simulink model "E020_R1_U2_aU_window_from_ideal_iqcot_20260701_144800"  (R2024b)
settings: Solver=VariableStepAuto  StartTime=0.0  StopTime=0.54e-3  MaxStep=5e-9  RelTol=1e-3
undefined symbols (not defined in the file): A_init, A_lower, A_upper, Cout, DCR_L1, DCR_L2, DCR_L3, DCR_L4, E020_Boost_Decay_Rate, E020_CurrentLimit_Guard, E020_FastRequest_Enable, E020_FastRequest_Period, E020_FastRequest_PulseWidth, E020_FastRequest_Window, E020_LateRecoveryGuard_Enable, E020_Settling_Band, E020_TonBoost_Enable, E020_TonBoost_Window, E020_Undershoot_Band, E020_Vref, ESR_C, IdealIQCOT_Enable, IL_adc_counts_per_A, IL_pk_limit_adc_neg, IL_pk_limit_adc_pos, Iload_final, Iload_initial, Iph, Iqcot_enable, kappa_cmd, Kiqcot, Kvc_iqcot, L, Lambda0_iqcot, Lambda_m2, rho_cmd, Ri_iqcot, t_load_step, Tblank, Tdead, Tiqcot_leak, Toff_min, Ton_cmd, Ton_iq_max, Ton_iq_min, Ts_ctrl, Tslot, Tss, Tton_boost_max, Vc_bias_iqcot, Vcot_ramp_amp, Vcot_ramp_enable, Vhys, Vin, Vo_ref
libraries: simulink x29, spsCurrentMeasurementLib x8, spsMosfetLib x8, spsSeriesRLCBranchLib x5, spsVoltageMeasurementLib x5, spsDCVoltageSourceLib x4, spsControlledCurrentSourceLib x1, spsGroundLib x1, spspowerguiLib x1
(part 2 of 2)

== system E020_R1_U2_aU_window_from_ideal_iqcot_20260701_144800/GateDriver_1Phase1/OnDelay1 ==
  u : Inport
  Compare To Constant : simulink/Logic and Bit Operations/Compare To Constant  relop=>=  const=Tdead  OutDataTypeStr=boolean
  Data Type Conversion : DataTypeConversion  OutDataTypeStr=double  SaturateOnIntegerOverflow=off  RndMeth=Floor
  Integrator : Integrator  ExternalReset=level
  Logical Operator : Logic  Operator=NOT  AllPortsSameDT=off  OutDataTypeStr=boolean
  y : Outport
  wires:
  u/1 -> Data Type Conversion/1, Logical Operator/1
  Logical Operator/1 -> Integrator/2
  Data Type Conversion/1 -> Integrator/1
  Integrator/1 -> Compare To Constant/1
  Compare To Constant/1 -> y/1

== system E020_R1_U2_aU_window_from_ideal_iqcot_20260701_144800/GateDriver_1Phase2/OnDelay ==
  u : Inport
  Compare To Constant : simulink/Logic and Bit Operations/Compare To Constant  relop=>=  const=Tdead  OutDataTypeStr=boolean
  Data Type Conversion : DataTypeConversion  OutDataTypeStr=double  SaturateOnIntegerOverflow=off  RndMeth=Floor
  Integrator : Integrator  ExternalReset=level
  Logical Operator : Logic  Operator=NOT  AllPortsSameDT=off  OutDataTypeStr=boolean
  y : Outport
  wires:
  u/1 -> Data Type Conversion/1, Logical Operator/1
  Logical Operator/1 -> Integrator/2
  Data Type Conversion/1 -> Integrator/1
  Integrator/1 -> Compare To Constant/1
  Compare To Constant/1 -> y/1

== system E020_R1_U2_aU_window_from_ideal_iqcot_20260701_144800/GateDriver_1Phase2/OnDelay1 ==
  u : Inport
  Compare To Constant : simulink/Logic and Bit Operations/Compare To Constant  relop=>=  const=Tdead  OutDataTypeStr=boolean
  Data Type Conversion : DataTypeConversion  OutDataTypeStr=double  SaturateOnIntegerOverflow=off  RndMeth=Floor
  Integrator : Integrator  ExternalReset=level
  Logical Operator : Logic  Operator=NOT  AllPortsSameDT=off  OutDataTypeStr=boolean
  y : Outport
  wires:
  u/1 -> Data Type Conversion/1, Logical Operator/1
  Logical Operator/1 -> Integrator/2
  Data Type Conversion/1 -> Integrator/1
  Integrator/1 -> Compare To Constant/1
  Compare To Constant/1 -> y/1

== system E020_R1_U2_aU_window_from_ideal_iqcot_20260701_144800/GateDriver_1Phase3/OnDelay ==
  u : Inport
  Compare To Constant : simulink/Logic and Bit Operations/Compare To Constant  relop=>=  const=Tdead  OutDataTypeStr=boolean
  Data Type Conversion : DataTypeConversion  OutDataTypeStr=double  SaturateOnIntegerOverflow=off  RndMeth=Floor
  Integrator : Integrator  ExternalReset=level
  Logical Operator : Logic  Operator=NOT  AllPortsSameDT=off  OutDataTypeStr=boolean
  y : Outport
  wires:
  u/1 -> Data Type Conversion/1, Logical Operator/1
  Logical Operator/1 -> Integrator/2
  Data Type Conversion/1 -> Integrator/1
  Integrator/1 -> Compare To Constant/1
  Compare To Constant/1 -> y/1

== system E020_R1_U2_aU_window_from_ideal_iqcot_20260701_144800/GateDriver_1Phase3/OnDelay1 ==
  u : Inport
  Compare To Constant : simulink/Logic and Bit Operations/Compare To Constant  relop=>=  const=Tdead  OutDataTypeStr=boolean
  Data Type Conversion : DataTypeConversion  OutDataTypeStr=double  SaturateOnIntegerOverflow=off  RndMeth=Floor
  Integrator : Integrator  ExternalReset=level
  Logical Operator : Logic  Operator=NOT  AllPortsSameDT=off  OutDataTypeStr=boolean
  y : Outport
  wires:
  u/1 -> Data Type Conversion/1, Logical Operator/1
  Logical Operator/1 -> Integrator/2
  Data Type Conversion/1 -> Integrator/1
  Integrator/1 -> Compare To Constant/1
  Compare To Constant/1 -> y/1

== system E020_R1_U2_aU_window_from_ideal_iqcot_20260701_144800/GateDriver_1Phase4/OnDelay ==
  u : Inport
  Compare To Constant : simulink/Logic and Bit Operations/Compare To Constant  relop=>=  const=Tdead  OutDataTypeStr=boolean
  Data Type Conversion : DataTypeConversion  OutDataTypeStr=double  SaturateOnIntegerOverflow=off  RndMeth=Floor
  Integrator : Integrator  ExternalReset=level
  Logical Operator : Logic  Operator=NOT  AllPortsSameDT=off  OutDataTypeStr=boolean
  y : Outport
  wires:
  u/1 -> Data Type Conversion/1, Logical Operator/1
  Logical Operator/1 -> Integrator/2
  Data Type Conversion/1 -> Integrator/1
  Integrator/1 -> Compare To Constant/1
  Compare To Constant/1 -> y/1

== system E020_R1_U2_aU_window_from_ideal_iqcot_20260701_144800/GateDriver_1Phase4/OnDelay1 ==
  u : Inport
  Compare To Constant : simulink/Logic and Bit Operations/Compare To Constant  relop=>=  const=Tdead  OutDataTypeStr=boolean
  Data Type Conversion : DataTypeConversion  OutDataTypeStr=double  SaturateOnIntegerOverflow=off  RndMeth=Floor
  Integrator : Integrator  ExternalReset=level
  Logical Operator : Logic  Operator=NOT  AllPortsSameDT=off  OutDataTypeStr=boolean
  y : Outport
  wires:
  u/1 -> Data Type Conversion/1, Logical Operator/1
  Logical Operator/1 -> Integrator/2
  Data Type Conversion/1 -> Integrator/1
  Integrator/1 -> Compare To Constant/1
  Compare To Constant/1 -> y/1

== matlab function E020_R1_U2_aU_window_from_ideal_iqcot_20260701_144800/E020_TonBoost1 ==
  data: ton_in input double size=1; ton_out output double size=1; t input double size=1; t_step input double size=1; t_window input double size=1; t_max input double size=1; decay_rate input double size=1; enable input double size=1; vout input double size=1; vref input double size=1; band input double size=1; il_i input double size=1; current_limit input double size=1; late_guard_enable input double size=1; target_load input double size=1; settle_band input double size=1; il1 input double size=1; il2 input double size=1; il3 input double size=1; il4 input double size=1; boost_active output double size=1; boost_state output double size=1; boost_gain output double size=1; boost_window output double size=1; boost_decay_state output double size=1; fallback_state output double size=1
function [ton_out,boost_active,boost_state,boost_gain,boost_window,boost_decay_state,fallback_state] = ton_boost(ton_in,t,t_step,t_window,t_max,decay_rate,enable,vout,vref,band,il_i,current_limit,late_guard_enable,target_load,settle_band,il1,il2,il3,il4)
%#codegen
persistent prev_t prev_error
if isempty(prev_t)
    prev_t = t;
end
if isempty(prev_error)
    prev_error = vout - vref;
end
age = t - t_step;
in_window = (enable > 0.5) && (age >= 0.0) && (age <= t_window);
deficit = vout <= (vref - band);
guard_ok = (current_limit <= 0.0) || (abs(il_i) <= current_limit);
verr = vout - vref;
dt = max(t - prev_t, eps);
verr_slope = (verr - prev_error) / dt;
current_target_reached = (t >= t_step) && ((il1 + il2 + il3 + il4) >= 0.9 * target_load);
slope_release = (verr < 0.0) && (verr_slope > 0.0);
band_release = abs(verr) <= max(5.0 * settle_band, settle_band);
late_guard = (late_guard_enable > 0.5) && (t >= t_step) && (current_target_reached || slope_release || band_release);
active = in_window && deficit && guard_ok && ~late_guard && (t_max > ton_in);
boost_window = t_window;
boost_gain = 0.0;
boost_decay_state = 0.0;
if active
    decay = exp(-max(decay_rate, 0.0) * max(age, 0.0));
    target = ton_in + (t_max - ton_in) * decay;
    ton_out = min(max(target, ton_in), t_max);
    boost_gain = decay;
    boost_decay_state = double(decay < 0.1);
else
    ton_out = ton_in;
end
boost_active = double(active);
boost_state = double(in_window && deficit && guard_ok && ~late_guard);
fallback_state = double((t >= t_step) && ((~active && age > t_window) || late_guard));
prev_t = t;
prev_error = verr;

== matlab function E020_R1_U2_aU_window_from_ideal_iqcot_20260701_144800/E020_TonBoost2 ==
  data: ton_in input double size=1; ton_out output double size=1; t input double size=1; t_step input double size=1; t_window input double size=1; t_max input double size=1; decay_rate input double size=1; enable input double size=1; vout input double size=1; vref input double size=1; band input double size=1; il_i input double size=1; current_limit input double size=1; late_guard_enable input double size=1; target_load input double size=1; settle_band input double size=1; il1 input double size=1; il2 input double size=1; il3 input double size=1; il4 input double size=1; boost_active output double size=1; boost_state output double size=1; boost_gain output double size=1; boost_window output double size=1; boost_decay_state output double size=1; fallback_state output double size=1
function [ton_out,boost_active,boost_state,boost_gain,boost_window,boost_decay_state,fallback_state] = ton_boost(ton_in,t,t_step,t_window,t_max,decay_rate,enable,vout,vref,band,il_i,current_limit,late_guard_enable,target_load,settle_band,il1,il2,il3,il4)
%#codegen
persistent prev_t prev_error
if isempty(prev_t)
    prev_t = t;
end
if isempty(prev_error)
    prev_error = vout - vref;
end
age = t - t_step;
in_window = (enable > 0.5) && (age >= 0.0) && (age <= t_window);
deficit = vout <= (vref - band);
guard_ok = (current_limit <= 0.0) || (abs(il_i) <= current_limit);
verr = vout - vref;
dt = max(t - prev_t, eps);
verr_slope = (verr - prev_error) / dt;
current_target_reached = (t >= t_step) && ((il1 + il2 + il3 + il4) >= 0.9 * target_load);
slope_release = (verr < 0.0) && (verr_slope > 0.0);
band_release = abs(verr) <= max(5.0 * settle_band, settle_band);
late_guard = (late_guard_enable > 0.5) && (t >= t_step) && (current_target_reached || slope_release || band_release);
active = in_window && deficit && guard_ok && ~late_guard && (t_max > ton_in);
boost_window = t_window;
boost_gain = 0.0;
boost_decay_state = 0.0;
if active
    decay = exp(-max(decay_rate, 0.0) * max(age, 0.0));
    target = ton_in + (t_max - ton_in) * decay;
    ton_out = min(max(target, ton_in), t_max);
    boost_gain = decay;
    boost_decay_state = double(decay < 0.1);
else
    ton_out = ton_in;
end
boost_active = double(active);
boost_state = double(in_window && deficit && guard_ok && ~late_guard);
fallback_state = double((t >= t_step) && ((~active && age > t_window) || late_guard));
prev_t = t;
prev_error = verr;

== matlab function E020_R1_U2_aU_window_from_ideal_iqcot_20260701_144800/E020_TonBoost3 ==
  data: ton_in input double size=1; ton_out output double size=1; t input double size=1; t_step input double size=1; t_window input double size=1; t_max input double size=1; decay_rate input double size=1; enable input double size=1; vout input double size=1; vref input double size=1; band input double size=1; il_i input double size=1; current_limit input double size=1; late_guard_enable input double size=1; target_load input double size=1; settle_band input double size=1; il1 input double size=1; il2 input double size=1; il3 input double size=1; il4 input double size=1; boost_active output double size=1; boost_state output double size=1; boost_gain output double size=1; boost_window output double size=1; boost_decay_state output double size=1; fallback_state output double size=1
function [ton_out,boost_active,boost_state,boost_gain,boost_window,boost_decay_state,fallback_state] = ton_boost(ton_in,t,t_step,t_window,t_max,decay_rate,enable,vout,vref,band,il_i,current_limit,late_guard_enable,target_load,settle_band,il1,il2,il3,il4)
%#codegen
persistent prev_t prev_error
if isempty(prev_t)
    prev_t = t;
end
if isempty(prev_error)
    prev_error = vout - vref;
end
age = t - t_step;
in_window = (enable > 0.5) && (age >= 0.0) && (age <= t_window);
deficit = vout <= (vref - band);
guard_ok = (current_limit <= 0.0) || (abs(il_i) <= current_limit);
verr = vout - vref;
dt = max(t - prev_t, eps);
verr_slope = (verr - prev_error) / dt;
current_target_reached = (t >= t_step) && ((il1 + il2 + il3 + il4) >= 0.9 * target_load);
slope_release = (verr < 0.0) && (verr_slope > 0.0);
band_release = abs(verr) <= max(5.0 * settle_band, settle_band);
late_guard = (late_guard_enable > 0.5) && (t >= t_step) && (current_target_reached || slope_release || band_release);
active = in_window && deficit && guard_ok && ~late_guard && (t_max > ton_in);
boost_window = t_window;
boost_gain = 0.0;
boost_decay_state = 0.0;
if active
    decay = exp(-max(decay_rate, 0.0) * max(age, 0.0));
    target = ton_in + (t_max - ton_in) * decay;
    ton_out = min(max(target, ton_in), t_max);
    boost_gain = decay;
    boost_decay_state = double(decay < 0.1);
else
    ton_out = ton_in;
end
boost_active = double(active);
boost_state = double(in_window && deficit && guard_ok && ~late_guard);
fallback_state = double((t >= t_step) && ((~active && age > t_window) || late_guard));
prev_t = t;
prev_error = verr;

== matlab function E020_R1_U2_aU_window_from_ideal_iqcot_20260701_144800/E020_TonBoost4 ==
  data: ton_in input double size=1; ton_out output double size=1; t input double size=1; t_step input double size=1; t_window input double size=1; t_max input double size=1; decay_rate input double size=1; enable input double size=1; vout input double size=1; vref input double size=1; band input double size=1; il_i input double size=1; current_limit input double size=1; late_guard_enable input double size=1; target_load input double size=1; settle_band input double size=1; il1 input double size=1; il2 input double size=1; il3 input double size=1; il4 input double size=1; boost_active output double size=1; boost_state output double size=1; boost_gain output double size=1; boost_window output double size=1; boost_decay_state output double size=1; fallback_state output double size=1
function [ton_out,boost_active,boost_state,boost_gain,boost_window,boost_decay_state,fallback_state] = ton_boost(ton_in,t,t_step,t_window,t_max,decay_rate,enable,vout,vref,band,il_i,current_limit,late_guard_enable,target_load,settle_band,il1,il2,il3,il4)
%#codegen
persistent prev_t prev_error
if isempty(prev_t)
    prev_t = t;
end
if isempty(prev_error)
    prev_error = vout - vref;
end
age = t - t_step;
in_window = (enable > 0.5) && (age >= 0.0) && (age <= t_window);
deficit = vout <= (vref - band);
guard_ok = (current_limit <= 0.0) || (abs(il_i) <= current_limit);
verr = vout - vref;
dt = max(t - prev_t, eps);
verr_slope = (verr - prev_error) / dt;
current_target_reached = (t >= t_step) && ((il1 + il2 + il3 + il4) >= 0.9 * target_load);
slope_release = (verr < 0.0) && (verr_slope > 0.0);
band_release = abs(verr) <= max(5.0 * settle_band, settle_band);
late_guard = (late_guard_enable > 0.5) && (t >= t_step) && (current_target_reached || slope_release || band_release);
active = in_window && deficit && guard_ok && ~late_guard && (t_max > ton_in);
boost_window = t_window;
boost_gain = 0.0;
boost_decay_state = 0.0;
if active
    decay = exp(-max(decay_rate, 0.0) * max(age, 0.0));
    target = ton_in + (t_max - ton_in) * decay;
    ton_out = min(max(target, ton_in), t_max);
    boost_gain = decay;
    boost_decay_state = double(decay < 0.1);
else
    ton_out = ton_in;
end
boost_active = double(active);
boost_state = double(in_window && deficit && guard_ok && ~late_guard);
fallback_state = double((t >= t_step) && ((~active && age > t_window) || late_guard));
prev_t = t;
prev_error = verr;

== matlab function E020_R1_U2_aU_window_from_ideal_iqcot_20260701_144800/E020_TonActual1 ==
  data: qh input boolean size=1; Ton_actual output double size=1; t input double size=1
function Ton_actual = ton_actual_estimator(qh, t)
%#codegen
persistent q_prev t_rise last_width
if isempty(q_prev)
    q_prev = 0.0;
end
if isempty(t_rise)
    t_rise = 0.0;
end
if isempty(last_width)
    last_width = 0.0;
end
is_high = double(qh > 0.5);
if is_high > 0.5 && q_prev <= 0.5
    t_rise = t;
elseif is_high <= 0.5 && q_prev > 0.5
    last_width = max(0.0, t - t_rise);
end
Ton_actual = last_width;
q_prev = is_high;

== matlab function E020_R1_U2_aU_window_from_ideal_iqcot_20260701_144800/E020_TonActual2 ==
  data: qh input boolean size=1; Ton_actual output double size=1; t input double size=1
function Ton_actual = ton_actual_estimator(qh, t)
%#codegen
persistent q_prev t_rise last_width
if isempty(q_prev)
    q_prev = 0.0;
end
if isempty(t_rise)
    t_rise = 0.0;
end
if isempty(last_width)
    last_width = 0.0;
end
is_high = double(qh > 0.5);
if is_high > 0.5 && q_prev <= 0.5
    t_rise = t;
elseif is_high <= 0.5 && q_prev > 0.5
    last_width = max(0.0, t - t_rise);
end
Ton_actual = last_width;
q_prev = is_high;

== matlab function E020_R1_U2_aU_window_from_ideal_iqcot_20260701_144800/E020_TonActual3 ==
  data: qh input boolean size=1; Ton_actual output double size=1; t input double size=1
function Ton_actual = ton_actual_estimator(qh, t)
%#codegen
persistent q_prev t_rise last_width
if isempty(q_prev)
    q_prev = 0.0;
end
if isempty(t_rise)
    t_rise = 0.0;
end
if isempty(last_width)
    last_width = 0.0;
end
is_high = double(qh > 0.5);
if is_high > 0.5 && q_prev <= 0.5
    t_rise = t;
elseif is_high <= 0.5 && q_prev > 0.5
    last_width = max(0.0, t - t_rise);
end
Ton_actual = last_width;
q_prev = is_high;

== matlab function E020_R1_U2_aU_window_from_ideal_iqcot_20260701_144800/E020_TonActual4 ==
  data: qh input boolean size=1; Ton_actual output double size=1; t input double size=1
function Ton_actual = ton_actual_estimator(qh, t)
%#codegen
persistent q_prev t_rise last_width
if isempty(q_prev)
    q_prev = 0.0;
end
if isempty(t_rise)
    t_rise = 0.0;
end
if isempty(last_width)
    last_width = 0.0;
end
is_high = double(qh > 0.5);
if is_high > 0.5 && q_prev <= 0.5
    t_rise = t;
elseif is_high <= 0.5 && q_prev > 0.5
    last_width = max(0.0, t - t_rise);
end
Ton_actual = last_width;
q_prev = is_high;

== matlab function E020_R1_U2_aU_window_from_ideal_iqcot_20260701_144800/E020_R1_Diagnostic ==
  data: t input double size=1; current_limit_hit output double size=1; vout input double size=1; vref input double size=1; t_step input double size=1; target_load input double size=1; current_limit input double size=1; settle_band input double size=1; late_guard_enable input double size=1; il1 input double size=1; il2 input double size=1; il3 input double size=1; il4 input double size=1; phase_current_peak output double size=1; current_rise_target_state output double size=1; late_recovery_guard_state output double size=1; Vout_error output double size=1; Vout_error_slope output double size=1; settling_band_state output double size=1; phase_order_error output double size=1; REQ_reject_reason output double size=1
function [current_limit_hit,phase_current_peak,current_rise_target_state,late_recovery_guard_state,Vout_error,Vout_error_slope,settling_band_state,phase_order_error,REQ_reject_reason] = r1_diag(t,vout,vref,t_step,target_load,current_limit,settle_band,late_guard_enable,il1,il2,il3,il4)
%#codegen
persistent prev_t prev_error
if isempty(prev_t)
    prev_t = t;
end
if isempty(prev_error)
    prev_error = vout - vref;
end
Vout_error = vout - vref;
dt = max(t - prev_t, eps);
Vout_error_slope = (Vout_error - prev_error) / dt;
phase_current_peak = max(max(abs(il1), abs(il2)), max(abs(il3), abs(il4)));
current_limit_hit = double((current_limit > 0.0) && (phase_current_peak > current_limit));
current_rise_target_state = double((t >= t_step) && ((il1 + il2 + il3 + il4) >= 0.9 * target_load));
settling_band_state = double(abs(Vout_error) <= settle_band);
slope_release = (Vout_error < 0.0) && (Vout_error_slope > 0.0);
band_release = abs(Vout_error) <= max(5.0 * settle_band, settle_band);
late_recovery_guard_state = double((late_guard_enable > 0.5) && (t >= t_step) && (current_rise_target_state > 0.5 || slope_release || band_release));
phase_order_error = 0.0;
REQ_reject_reason = 0.0;
prev_t = t;
prev_error = Vout_error;

== matlab function E020_R1_U2_aU_window_from_ideal_iqcot_20260701_144800/Ideal_Digital_IQCOT_Request/IQCOT_Event_Core ==
  data: e_v input double size=1; REQ_iqcot output double size=1; IL1 input double size=1; IL2 input double size=1; IL3 input double size=1; IL4 input double size=1; phase_idx input double size=1; tr_reset input double size=1; enable input double size=1; Ts_ctrl_in input double size=1; Lambda0_in input double size=1; Lambda_m2_in input double size=1; rho_cmd_in input double size=1; Ri_in input double size=1; Kvc_in input double size=1; Vc_bias_in input double size=1; kappa_cmd_in input double size=1; A_init_in input double size=1; A_lower_in input double size=1; A_upper_in input double size=1; A_iqcot output double size=1; Lambda_i output double size=1; h_iqcot output double size=1; IL_sel output double size=1; vc_ctrl output double size=1
function [REQ_iqcot,A_iqcot,Lambda_i,h_iqcot,IL_sel,vc_ctrl] = IQCOT_Event_Core(e_v,IL1,IL2,IL3,IL4,phase_idx,tr_reset,enable,Ts_ctrl_in,Lambda0_in,Lambda_m2_in,rho_cmd_in,Ri_in,Kvc_in,Vc_bias_in,kappa_cmd_in,A_init_in,A_lower_in,A_upper_in)
%#codegen
REQ_iqcot = 0.0;
A_iqcot = 0.0;
Lambda_i = 0.0;
h_iqcot = 0.0;
IL_sel = 0.0;
vc_ctrl = 0.0;
persistent Astate reset_prev phase_prev
if isempty(Astate)
    Astate = double(A_init_in);
end
if isempty(reset_prev)
    reset_prev = 0.0;
end
if isempty(phase_prev)
    phase_prev = 0.0;
end
p = floor(double(phase_idx));
p = mod(p, 4);
if p == 0
    IL_sel = IL1;
elseif p == 1
    IL_sel = IL2;
elseif p == 2
    IL_sel = IL3;
else
    IL_sel = IL4;
end
Ri_eff = Ri_in * exp(kappa_cmd_in);
vc_ctrl = Vc_bias_in + Kvc_in * e_v;
h_iqcot = vc_ctrl - Ri_eff * IL_sel;
Lambda_i = Lambda0_in * (1 + rho_cmd_in) + Lambda_m2_in * cos(pi * p);
if Lambda_i < eps
    Lambda_i = eps;
end
A_update = Astate + Ts_ctrl_in * h_iqcot;
if A_update < A_lower_in
    A_update = A_lower_in;
end
if A_update > A_upper_in
    A_update = A_upper_in;
end
REQ_iqcot = double((enable > 0.5) && (A_update >= Lambda_i));
A_iqcot = A_update;
reset_rise = (tr_reset > 0.5) && (reset_prev <= 0.5);
phase_change = (p ~= phase_prev);
if enable <= 0.5
    Astate = A_init_in;
elseif reset_rise || phase_change
    Astate = A_init_in;
else
    Astate = A_update;
end
reset_prev = double(tr_reset);
phase_prev = p;

== matlab function E020_R1_U2_aU_window_from_ideal_iqcot_20260701_144800/E020_FastRequest ==
  data: tr_in input boolean size=1; tr_out output boolean size=1; t input double size=1; t_step input double size=1; t_window input double size=1; period input double size=1; pulse_width input double size=1; enable input double size=1; vout input double size=1; vref input double size=1; band input double size=1; current_limit input double size=1; il1 input double size=1; il2 input double size=1; il3 input double size=1; il4 input double size=1; fast_active output double size=1; fast_count output double size=1; fast_reject_reason output double size=1; fast_state output double size=1
function [tr_out,fast_active,fast_count,fast_reject_reason,fast_state] = fast_request(tr_in,t,t_step,t_window,period,pulse_width,enable,vout,vref,band,current_limit,il1,il2,il3,il4)
%#codegen
base_tr = logical(tr_in);
age = t - t_step;
in_window = (enable > 0.5) && (age >= 0.0) && (age <= t_window);
deficit = vout <= (vref - band);
iph_peak = max(max(abs(il1), abs(il2)), max(abs(il3), abs(il4)));
guard_ok = (current_limit <= 0.0) || (iph_peak <= current_limit);
pulse = false;
if in_window && deficit && guard_ok && (period > 0.0) && (pulse_width > 0.0)
    slot = age - floor(age / period) * period;
    pulse = slot <= min(pulse_width, period);
end
fast_reject_reason = 0.0;
if enable <= 0.5
    fast_reject_reason = 1.0;
elseif age < 0.0 || age > t_window
    fast_reject_reason = 2.0;
elseif ~deficit
    fast_reject_reason = 3.0;
elseif ~guard_ok
    fast_reject_reason = 4.0;
elseif period <= 0.0 || pulse_width <= 0.0
    fast_reject_reason = 5.0;
end
tr_out = base_tr || pulse;
fast_active = double(pulse && ~base_tr);
fast_count = fast_active;
fast_state = double(in_window && deficit && guard_ok);
